simulink model "sgMdl_IO755_IO756_EthernetIPLoopback"  (R2024b)
settings: Solver=FixedStepAuto  StartTime=0.0  StopTime=inf  RelTol=1e-3  EnableMultiTasking=on
undefined symbols (not defined in the file): C, Ts
libraries: slrealtimeutilitieslib x4, speedgoatlib_IO755 x3, speedgoatlib_IO756 x3, simulink x2, speedgoatlib_shared x2
Description:
  | IO755 & IO756 - Ethernet/IP Loopback
settings Model: ModifiedByFormat=Speedgoat  Creator=Speedgoat  LastModifiedBy=Speedgoat
settings SolverCC: ConcurrentTasks=on  AlgebraicLoopSolver=TrustRegion  PositivePriorityOrder=on  AutoInsertRateTranBlk=on  InsertRTBMode=Never (minimum delay)
settings DataIOCC: SaveFormat=Array  SaveState=on  SignalLoggingName=logsOut
settings OptimizationCC: BlockReduction=off  BooleanDataType=off  OptimizeBlockIOStorage=off  BufferReuse=off  GlobalBufferReuse=off  ExpressionFolding=off  LocalBlockOutputs=off  InitFltsAndDblsToZero=on  OptimizeDataStoreBuffers=off  BusAssignmentInplaceUpdate=off
settings DebuggingCC: SaveWithParameterizedLinksMsg=none  UnderspecifiedInitializationDetection=Classic  MergeDetectMultiDrivingBlocksExec=none  CheckExecutionContextPreStartOutputMsg=on  SignalResolutionControl=TryResolveAllWithWarning  TasksWithSamePriorityMsg=none  UnconnectedInputMsg=warning  UnconnectedOutputMsg=warning  UnconnectedLineMsg=warning  SFUnexpectedBacktrackingDiag=warning  SFNoUnconditionalDefaultTransitionDiag=warning  SFExecutionAtInitializationDiag=none  ArithmeticOperatorsInVariantConditions=warning
settings HardwareCC: ProdBitPerLong=64  ProdLongLongMode=on  ProdHWDeviceType=Intel->x86-64 (Linux 64)
settings ModelReferenceCC: EnableRefExpFcnMdlSchedulingChecks=on  PropagateSignalLabelsOutOfModel=off
settings SFSimCC: SimUseLocalCustomCode=off  SimTargetLang=C++
settings RTWCC: Description=Speedgoat Real-Time Target Machine  SystemTargetFile=speedgoat.tlc  TemplateMakefile=slrealtime_default_tmf  RTWUseLocalCustomCode=off  Toolchain=Simulink Real-Time Toolchain  BuildConfiguration=Faster Runs  TargetLang=C++  GPUComputeCapability=3.5  DLArmComputeVersion=19.05
settings CodeAppCC: StateflowObjectComments=on
settings SimulinkRealTimeTargetCC: SubcomponentCodeInterfacePackaging=Reusable function  MATLABClassNameForMDSCustomization=Simulink.SoftwareTarget.GRTCustomization  InstructionSetFMA=off  LogToMDFFile=off  SLRTFileLogMaxRuns=10  UseGCCFastMath=on
settings ConfigComp: CovMetricSettings=dw  CovSaveCumulativeToWorkspaceVar=on  CovSaveSingleToWorkspaceVar=on  CovExternalEMLEnable=off  CovSFcnEnable=off  CovBoundaryAbsTol=1.0e-5

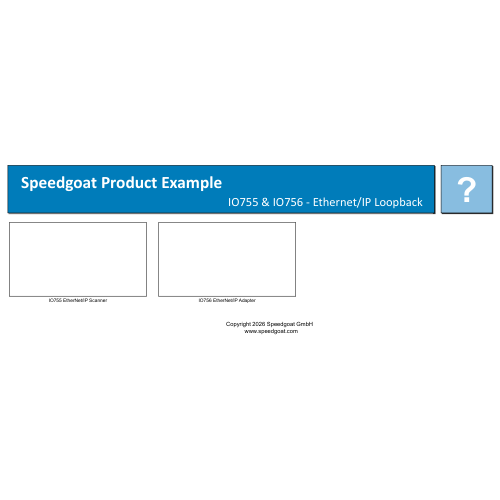
[thumbnail: Simulink's stored preview of the top-level diagram]
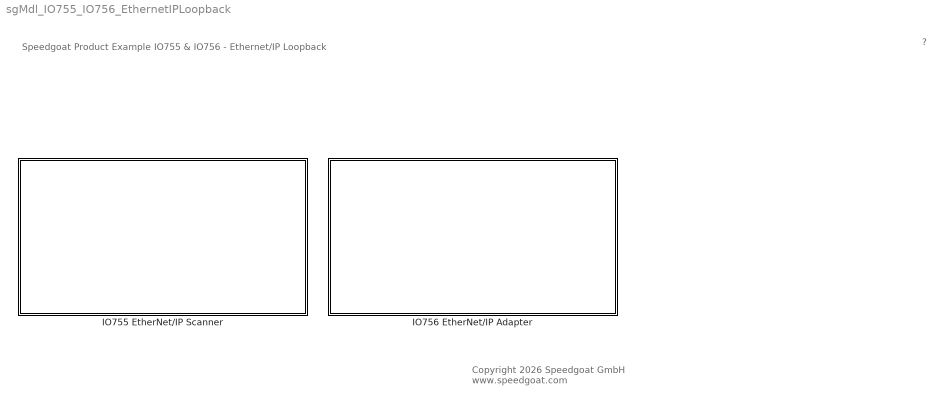
== system sgMdl_IO755_IO756_EthernetIPLoopback ==
  note: Speedgoat Product Example
      | IO755 & IO756 - Ethernet/IP Loopback
  note: ?
  note: Copyright 2026 Speedgoat GmbH
      |  www.speedgoat.com
  IO755 EtherNet/IP Scanner : Subsystem
  IO756 EtherNet/IP Adapter : Subsystem

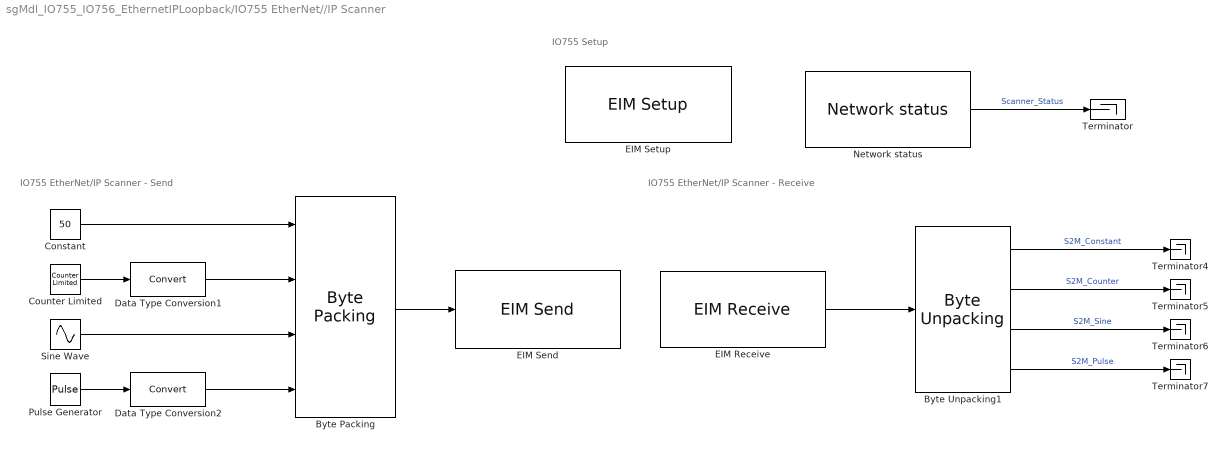
== system sgMdl_IO755_IO756_EthernetIPLoopback/IO755 EtherNet//IP Scanner ==
  note: IO755 EtherNet/IP Scanner - Receive
  note: IO755 EtherNet/IP Scanner - Send
  note: IO755 Setup
  Byte Packing : slrealtimeutilitieslib/Byte Packing  MaskPackedDataType=uint8  MaskUnpackedDataTypes={'int8','uint16','double','int32'}  MaskAlignment=1
  Byte Unpacking1 : slrealtimeutilitieslib/Byte Unpacking  MaskUnpackedDataTypes={'int16','uint32','single','uint8'}  MaskUnpackedDataSizes={[1],[1],[1],[1]}  MaskAlignment=1
  Constant : Constant  Value=50  OutDataTypeStr=Inherit: Inherit via back propagation  SampleTime=Ts
  Counter Limited : simulink/Sources/Counter Limited  uplimit=100  tsamp=Ts/Ts/10
  Data Type Conversion1 : DataTypeConversion  SaturateOnIntegerOverflow=off  RndMeth=Floor
  Data Type Conversion2 : DataTypeConversion  SaturateOnIntegerOverflow=off  RndMeth=Floor
  EIM Receive : speedgoatlib_IO755/EIM Receive  id=1  port_type=1 port with n element vector of type UINT8  in_address=0  in_length=11  ts=Ts  slot=0
      settings: SourceProductName=IO755 EtherNet/IP Scanner
  EIM Send : speedgoatlib_IO755/EIM Send  id=1  port_type=1 port with n element vector of type UINT8  out_address=0  out_length=15  ts=Ts
      settings: SourceProductName=IO755 EtherNet/IP Scanner
  EIM Setup : speedgoatlib_IO755/EIM Setup  Priority=0  id=1  drive=C:  ts=-1  slot=-1  qtyMods=[1,0,0]  ConfigFile1=which('IO755_IO756_Loopback_m.nxd')  ConfigFile2=which('IO755_IO756_Loopback_m_nwid.nxd')  protocol=IO755  firmware=EtherNet/IP Scanner
      settings: SourceProductName=IO755 EtherNet/IP Scanner
  Network status : speedgoatlib_shared/IO75X/Network status  id=1  get_status=on  set_status=off  timeout=0.01  ts=Ts
  Pulse Generator : DiscretePulseGenerator  Amplitude=100  Period=2*1/Ts  PulseWidth=1/Ts  SampleTime=Ts
  Sine Wave : Sin  Amplitude=100  Frequency=2*pi  Phase=pi  SampleTime=Ts
  Terminator{,4..7} (5 alike) : Terminator
  wires:
  Sine Wave/1 -> Byte Packing/3
  Counter Limited/1 -> Data Type Conversion1/1
  Constant/1 -> Byte Packing/1
  Byte Unpacking1/1 -> Terminator4/1  "S2M_Constant"
  Byte Unpacking1/2 -> Terminator5/1  "S2M_Counter"
  Byte Unpacking1/3 -> Terminator6/1  "S2M_Sine"
  Byte Unpacking1/4 -> Terminator7/1  "S2M_Pulse"
  Data Type Conversion1/1 -> Byte Packing/2
  Data Type Conversion2/1 -> Byte Packing/4
  Pulse Generator/1 -> Data Type Conversion2/1
  Byte Packing/1 -> EIM Send/1
  EIM Receive/1 -> Byte Unpacking1/1
  Network status/1 -> Terminator/1  "Scanner_Status"

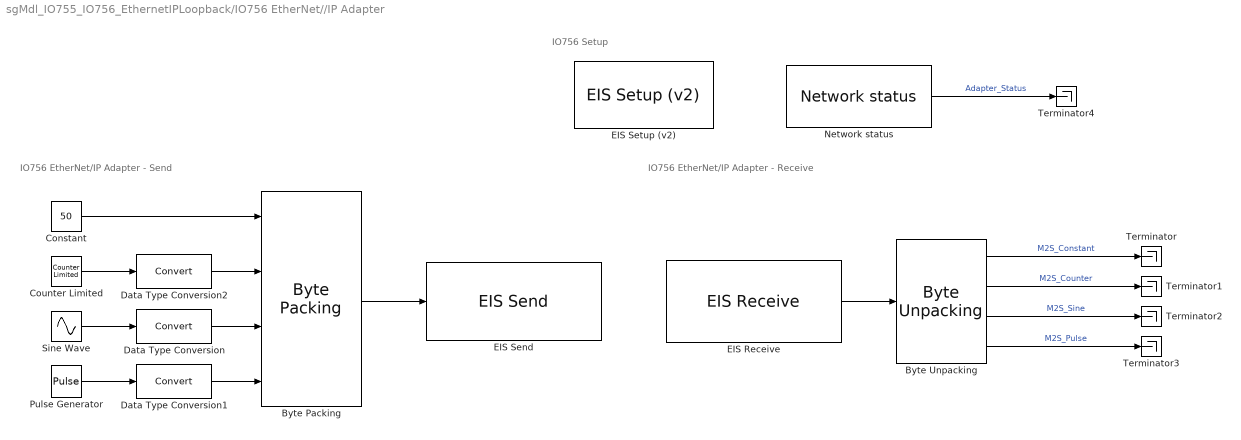
== system sgMdl_IO755_IO756_EthernetIPLoopback/IO756 EtherNet//IP Adapter ==
  note: IO756 Setup
  note: IO756 EtherNet/IP Adapter - Send
  note: IO756 EtherNet/IP Adapter - Receive
  Byte Packing : slrealtimeutilitieslib/Byte Packing  MaskPackedDataType=uint8  MaskUnpackedDataTypes={'int16','uint32','single','uint8'}  MaskAlignment=1
  Byte Unpacking : slrealtimeutilitieslib/Byte Unpacking  MaskUnpackedDataTypes={'int8','uint16','double','int32'}  MaskUnpackedDataSizes={[1],[1],[1],[1]}  MaskAlignment=1
  Constant : Constant  Value=50  OutDataTypeStr=Inherit: Inherit via back propagation  SampleTime=Ts
  Counter Limited : simulink/Sources/Counter Limited  uplimit=100  tsamp=Ts/Ts/10
  Data Type Conversion : DataTypeConversion  SaturateOnIntegerOverflow=off  RndMeth=Floor
  Data Type Conversion1 : DataTypeConversion  SaturateOnIntegerOverflow=off  RndMeth=Floor
  Data Type Conversion2 : DataTypeConversion  SaturateOnIntegerOverflow=off  RndMeth=Floor
  EIS Receive : speedgoatlib_IO756/EIS Receive  id=2  ts=Ts  parConfigMode=0  port_type=1 port with n element vector of type UINT8  in_length=15  parAssemblies=[]  parSetupBlockVersion=1
      settings: SourceProductName=IO756 EtherNet/IP Adapter
  EIS Send : speedgoatlib_IO756/EIS Send  id=2  ts=-1  parConfigMode=0  port_type=1 port with n element vector of type UINT8  out_length=11  parAssemblies=[]  parSetupBlockVersion=1
      settings: SourceProductName=IO756 EtherNet/IP Adapter
  EIS Setup (v2) : speedgoatlib_IO756/EIS Setup (v2)  parModuleId=2  parPciBusSlot=-1  parConfigMode=Simple  parIpAddress='192.168.10.2'  parNetmask='255.255.255.0'  parGateway='0.0.0.0'  parVendorId=283  parProductType=12  parProductCode=257  parMajorRev=1  parMinorRev=1  parDeviceName='CIFX RE/EIS'  parInputId=101  parInputLen=11  parInputFormat=Connection is pure data and is modeless  parOutputId=100  parOutputLen=15  parOutputFormat=32-bit run/idle header  parAssemblies=|  parConnections=[struct('InputID',101,'OutputID',100','ConfigID',0,'Type',0)]
      | [struct('ID',101,'Type','Output','Length',32,'Format',0), ...
      |  struct('ID',100,'Type','Input','Length',32,'Format',0)]
      settings: SourceProductName=IO756 EtherNet/IP Adapter
  Network status : speedgoatlib_shared/IO75X/Network status  id=2  get_status=on  set_status=off  timeout=0.01  ts=Ts
  Pulse Generator : DiscretePulseGenerator  Amplitude=100  Period=2*1/Ts  PulseWidth=1/Ts  SampleTime=Ts
  Sine Wave : Sin  Amplitude=100  Frequency=2*pi  Phase=pi  SampleTime=Ts
  Terminator{,1..4} (5 alike) : Terminator
  wires:
  EIS Receive/1 -> Byte Unpacking/1
  Byte Packing/1 -> EIS Send/1
  Byte Unpacking/1 -> Terminator/1  "M2S_Constant"
  Byte Unpacking/2 -> Terminator1/1  "M2S_Counter"
  Byte Unpacking/3 -> Terminator2/1  "M2S_Sine"
  Byte Unpacking/4 -> Terminator3/1  "M2S_Pulse"
  Constant/1 -> Byte Packing/1
  Counter Limited/1 -> Data Type Conversion2/1
  Sine Wave/1 -> Data Type Conversion/1
  Data Type Conversion/1 -> Byte Packing/3
  Data Type Conversion1/1 -> Byte Packing/4
  Data Type Conversion2/1 -> Byte Packing/2
  Pulse Generator/1 -> Data Type Conversion1/1
  Network status/1 -> Terminator4/1  "Adapter_Status"
